simulink model "my_sqrt"  (R2021b)
settings: Solver=FixedStepDiscrete  StartTime=0.0  StopTime=15  FixedStep=1  RelTol=1e-3
settings Model: Creator=francesco  LastModifiedBy=francesco

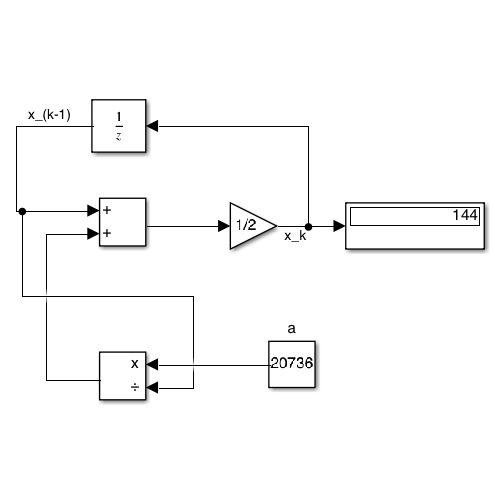
[thumbnail: Simulink's stored preview of the top-level diagram]
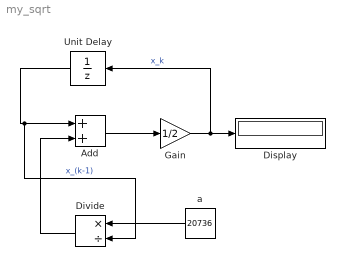
== system my_sqrt ==
  Add : Sum
  Display : Display
  Divide : Product  Inputs=*/
  Gain : Gain  Gain=1/2
  Unit Delay : UnitDelay  InitialCondition=0.2  SampleTime=-1  HasFrameUpgradeWarning=on
  a : Constant  Value=20736
  wires:
  Add/1 -> Gain/1
  Gain/1 -> Unit Delay/1, Display/1  "x_k"
  Unit Delay/1 -> Divide/2, Add/1  "x_(k-1)"
  a/1 -> Divide/1
  Divide/1 -> Add/2
